simulink model "Landing"  (R2019a)
settings: Solver=ode14x  StartTime=0.0  StopTime=141  FixedStep=1/30  MaxStep=0.02  RelTol=1e-3
undefined symbols (not defined in the file): airport_elevation, con_init, con_trim, glideslope, h_flare, h_RWY, init_x_pos, Ka, Kq, Psi_RWY, RWY_vector, SS_long, tau, Th23, trim_elevator, trim_thrust
libraries: simulink_extras x13, simulink x3, aerolibfltsims x2, cstblocks x1, aerolibanimutils x1, aerolibatmos2 x1
settings Model: Creator=tblaha  LastModifiedBy=tblaha

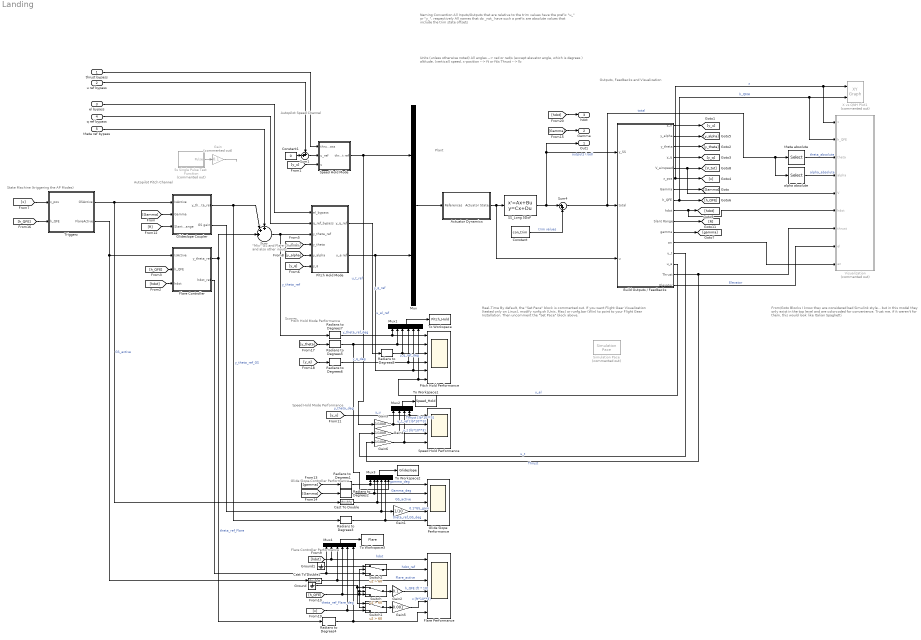
== system Landing ==
  note: Speed Hold Mode Performance
  note: Outputs, Feedbacks and Visualization
  note: Scopes
  note: Autopilot Speed Channel
  note: Autopilot Pitch Channel
  note: Plant
  note: State Machine (triggering the AP Modes)
  note: "Mix" GS and
      | Flare Channels
      | and also
      | other inputs
  note: Real-Time
      | By default, the "Set Pace" block is commented out.
      | If you want Flight Gear Visualization (tested only on Linux), modify runfg.sh (Unix, Mac) or runfg.bar (Win) to point to your Flight Gear Installation.
      | Then uncomment the "Set Pace" block above.
  note: From/Goto Blocks
      | I know they are considered bad Simulink style... but in this model they only exist in the top level and are colorcoded for convenience. Trust me, if it weren't for them, this would look like Italian Spaghetti
  note: Naming Convention
      | All Inputs/Outputs that are relative to the trim values have the prefix "u_" or "y_", respectively
      |
      | All names that do _not_ have such a prefix are absolute values that include the trim state offsets
  note: Units (unless otherwise noted)
      | All angles --> rad or rad/s (except elevator angle, which is degrees )
      | altitude, (vertical) speed, x-position --> ft or ft/s
      | Thrust --> lb
  note: Pitch Hold Mode Performance
  note: Flare Controller Performance
  note: Glide Slope Controller Performance
  thrust bypass : Inport
  u ref bypass : Inport  Port=2
  el bypass : Inport  Port=3
  q ref bypass : Inport  Port=4
  theta ref bypass : Inport  Port=5
  5s Single Pulse Test Function : Subsystem  Commented=on
  Actuator Dynamics : Subsystem
  Build Outputs / Feedbacks : Subsystem
  Cast To Double : DataTypeConversion  OutDataTypeStr=double
  Cast To Double1 : DataTypeConversion  OutDataTypeStr=double
  Constant : Constant  Value=con_trim
  Constant1 : Constant  Value=0
  Flare Controller : Subsystem
  Flare Performance : Scope  NumInputPorts=6
  Gain : Gain  Commented=on  Gain=0.1
  Gain1 : Gain  Gain=1/10
  Gain2 : Gain  Gain=0.1
  Gain3 : Gain  Gain=1/1000
  Gain4 : Gain  Gain=1/1000
  Gain5 : Gain  Gain=0.001
  Gain6 : Gain  Gain=1/1000
  Glide Slope Performance : Scope  NumInputPorts=5
  Glideslope Coupler : Subsystem
  Ground : Ground
  Ground1 : Ground
  Mux : Mux  Inputs=2
  Mux1 : Mux  Inputs=6
  Mux2 : Mux
  Mux3 : Mux  Inputs=6
  Mux4 : Mux  Inputs=6
  Pitch Hold Mode : Subsystem
  Pitch Hold Performance : Scope  NumInputPorts=6
  Radians to Degrees{1..8} (8 alike) : simulink_extras/Transformations/Radians to Degrees
  SS_Long 5DoF : StateSpace  A=SS_long.A  B=SS_long.B  C=SS_long.C  D=SS_long.D  InitialCondition=con_init
  Simulation Pace : aerolibanimutils/Simulation Pace  Commented=on  SimulationPace=1  SleepMode=Auto  OutputPaceError=off  SampleTime=1/30
  Speed Hold Mode : Subsystem
  Speed Hold Performance : Scope  NumInputPorts=4
  Sum : Sum  Inputs=+++||
  Sum1 : Sum  Inputs=++|
  Sum4 : Sum  Inputs=|++
  Switch : Switch  Criteria=u2 > Threshold  Threshold=60
  Switch1 : Switch  Criteria=u2 > Threshold  Threshold=60
  Switch2 : Switch  Criteria=u2 > Threshold  Threshold=60
  To Workspace : ToWorkspace  VariableName=Pitch_Hold  SampleTime=-1
  To Workspace1 : ToWorkspace  VariableName=Speed_Hold  SampleTime=-1
  To Workspace2 : ToWorkspace  VariableName=Glideslope  SampleTime=-1
  To Workspace3 : ToWorkspace  VariableName=Flare  SampleTime=-1
  Triggerz : Subsystem
  Visualization : Subsystem  Commented=on
  X vs QNH Plot1 : simulink/Sinks/XY Graph  Commented=on  xmin=-45000  xmax=5000  ymin=-100  ymax=2100  st=-1
  alpha absolute : Selector  InputPortWidth=5  IndexOptions=Index vector (dialog)  Indices=3  OutputSizes=1
  theta absolute : Selector  InputPortWidth=5  IndexOptions=Index vector (dialog)  Indices=4  OutputSizes=1
  Out1 : Outport
  Gamma : Outport  Port=2
  hdot : Outport  Port=3
  wires:
  Pitch Hold Mode/2(u_e ref) -> Mux/2, Mux1/5, Pitch Hold Performance/5  "u_el_ref"
  Speed Hold Mode/1(thrust ref) -> Mux/1, Gain3/1  "u_t_ref"
  [y_u] -> Speed Hold Mode/3(u)
  SS_Long 5DoF/1 -> Build Outputs / Feedbacks/1(y_SS), Out1/1, Sum4/1  "outputs (rad)"
  Build Outputs / Feedbacks/7(Gamma) -> [Gamma]
  Build Outputs / Feedbacks/11(gamma) -> [gamma]
  Build Outputs / Feedbacks/3(y_theta) -> [y_theta]
  Mux/1 -> Actuator Dynamics/1(References)
  Actuator Dynamics/1(Actuator States) -> SS_Long 5DoF/1, Build Outputs / Feedbacks/3(u)
  Build Outputs / Feedbacks/4(y_q) -> [y_q]
  Constant/1 -> Sum4/2  "trim values"
  Build Outputs / Feedbacks/1(y_u) -> [y_u]
  Build Outputs / Feedbacks/2(y_alpha) -> [y_alpha]
  Build Outputs / Feedbacks/10(Slant Range) -> [R]
  [x] -> Triggerz/1(x_pos)
  [h_QFE] -> Triggerz/2(h_QFE)
  [Gamma] -> Glideslope Coupler/2(Gamma)
  [R] -> Glideslope Coupler/3(SlantRange)
  Glideslope Coupler/1(y_theta_ref) -> Radians to Degrees3/1, Sum/2  "y_theta_ref_GS"
  [y_theta] -> Pitch Hold Mode/4(y_theta)
  [y_alpha] -> Pitch Hold Mode/5(y_alpha)
  [y_q] -> Pitch Hold Mode/6(y_q)
  [hdot] -> Flare Controller/3(hdot)
  [h_QFE] -> Flare Controller/2(h_QFE)
  5s Single Pulse Test Function/1(Pulse) -> Gain/1
  Build Outputs / Feedbacks/12(an) -> Visualization/9(an)
  alpha absolute/1 -> Visualization/4(alpha)  "alpha_absolute"
  Build Outputs / Feedbacks/9(hdot) -> Visualization/6(hdot), [hdot]
  Sum4/1 -> theta absolute/1, alpha absolute/1, Build Outputs / Feedbacks/2(total)  "total"
  theta absolute/1 -> Visualization/3(theta)  "theta_absolute"
  Build Outputs / Feedbacks/16(Elevator) -> Visualization/8(el)  "Elevator"
  Build Outputs / Feedbacks/8(h_QFE) -> [h_QFE], Visualization/2(h_QFE), X vs QNH Plot1/2  "h_QNH"
  Build Outputs / Feedbacks/15(Thrust) -> Gain6/1, Visualization/7(thrust)  "Thrust"
  Build Outputs / Feedbacks/5(V_airspeed) -> Visualization/5(V), [V_tot]
  Build Outputs / Feedbacks/6(x_pos) -> [x], Visualization/1(x), X vs QNH Plot1/1  "x"
  Pitch Hold Mode/1(y_q_ref) -> Radians to Degrees8/1  "y_q_ref"
  Radians to Degrees4/1 -> Flare Performance/6, Mux4/6  "theta_ref_Flare_deg"
  Radians to Degrees2/1 -> Mux3/2, Glide Slope Performance/2  "Gamma_deg"
  Flare Controller/1(y_theta_ref) -> Sum/3, Radians to Degrees4/1  "theta_ref_Flare"
  Gain1/1 -> Glide Slope Performance/4  "0.1*GS_gain"
  [y_q] -> Radians to Degrees6/1
  Radians to Degrees1/1 -> Glide Slope Performance/1, Mux3/1  "gamma_deg"
  [h_QFE] -> Switch1/2, Switch2/2, Switch/2, Switch/3, Mux4/4
  [Gamma] -> Radians to Degrees2/1
  Flare Controller/2(hdot_ref) -> Mux4/1, Switch2/3
  Build Outputs / Feedbacks/14(u_e) -> Mux1/6, Pitch Hold Performance/6  "u_el"
  [y_theta] -> Radians to Degrees5/1
  [gamma] -> Radians to Degrees1/1
  [hdot] -> Mux4/2, Flare Performance/1  "hdot"
  Radians to Degrees6/1 -> Mux1/4, Pitch Hold Performance/4  "y_q_deg"
  Triggerz/1(GSActive) -> Glideslope Coupler/1(IsActive), Cast To Double/1  "GS_active"
  Radians to Degrees7/1 -> Mux1/1, Pitch Hold Performance/1  "y_theta_ref_deg"
  Radians to Degrees5/1 -> Mux3/6, Mux1/2, Pitch Hold Performance/2  "y_theta_deg"
  Radians to Degrees8/1 -> Mux1/3, Pitch Hold Performance/3  "y_q_ref_deg"
  Triggerz/2(FlareActive) -> Flare Controller/1(IsActive), Cast To Double1/1
  Glideslope Coupler/2(GS gain) -> Gain1/1, Mux3/4
  Radians to Degrees3/1 -> Glide Slope Performance/5, Mux3/5  "theta_ref_GS_deg"
  theta ref bypass/1 -> Sum/1
  Build Outputs / Feedbacks/13(u_t) -> Gain4/1  "u_t"
  [y_u] -> Mux2/4, Speed Hold Performance/1  "y_u"
  Gain3/1 -> Mux2/1, Speed Hold Performance/2  "u_t_ref [lb*10**3]"
  Gain4/1 -> Speed Hold Performance/3, Mux2/2  "u_t [lb*10**3]"
  Gain6/1 -> Mux2/3, Speed Hold Performance/4  "Thrust [lb*10**3]"
  q ref bypass/1 -> Pitch Hold Mode/2(q_ref_bypass)
  el bypass/1 -> Pitch Hold Mode/1(el_bypass)
  Sum1/1 -> Speed Hold Mode/2(u_ref)
  u ref bypass/1 -> Sum1/1
  thrust bypass/1 -> Speed Hold Mode/1(thrust bypass)
  [Gamma] -> Gamma/1
  Sum/1 -> Radians to Degrees7/1, Pitch Hold Mode/3(y_theta_ref)  "y_theta_ref"
  Gain/1 -> ?
  [hdot] -> hdot/1
  Switch/1 -> Gain2/1
  Ground/1 -> Switch/1, Switch1/1
  Gain2/1 -> Flare Performance/4  "h_QFE [ft * 10]"
  Switch1/1 -> Gain5/1
  Gain5/1 -> Flare Performance/5  "x [ft*10**3]"
  [x] -> Switch1/3, Mux4/5
  Switch2/1 -> Flare Performance/2  "hdot_ref"
  Ground1/1 -> Switch2/1
  Constant1/1 -> Sum1/2
  Mux1/1 -> To Workspace/1
  Mux2/1 -> To Workspace1/1
  Mux3/1 -> To Workspace2/1
  Mux4/1 -> To Workspace3/1
  Cast To Double/1 -> Glide Slope Performance/3, Mux3/3  "GS_active"
  Cast To Double1/1 -> Flare Performance/3, Mux4/3  "Flare_active"

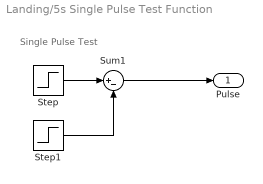
== system Landing/5s Single Pulse Test Function ==
  note: Single Pulse Test
  Step : Step  Time=5  SampleTime=0
  Step1 : Step  Time=10  SampleTime=0
  Sum1 : Sum  Inputs=|+-
  Pulse : Outport
  wires:
  Step/1 -> Sum1/1
  Step1/1 -> Sum1/2
  Sum1/1 -> Pulse/1

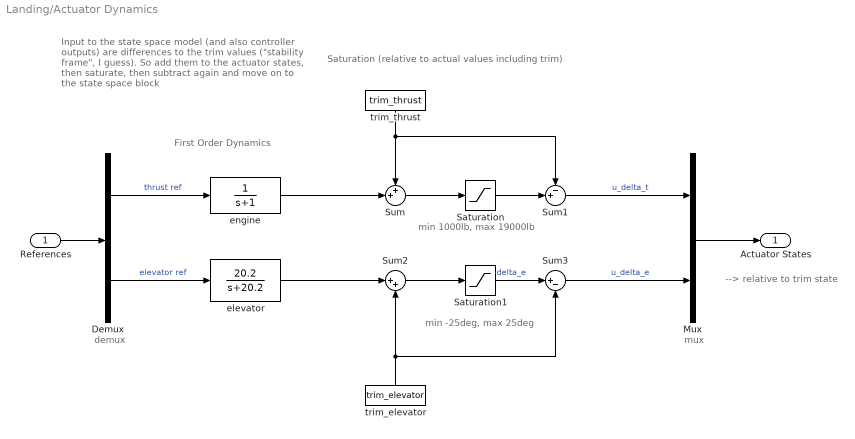
== system Landing/Actuator Dynamics ==
  note: --> relative to trim state
  note: Input to the state space model (and also controller outputs) are differences to the trim values ("stability frame", I guess). So add them to the actuator states, then saturate, then subtract again and move on to the state space block
  note: First Order Dynamics
  note: Saturation (relative to actual values including trim)
  note: demux
  note: min 1000lb, max 19000lb
  note: min -25deg, max 25deg
  note: mux
  References : Inport
  Demux : Demux  Outputs=2
  Mux : Mux  Inputs=2
  Saturation : Saturate  UpperLimit=19000  LowerLimit=1000
  Saturation1 : Saturate  UpperLimit=25  LowerLimit=-25
  Sum : Sum  Inputs=++|
  Sum1 : Sum  Inputs=-+|
  Sum2 : Sum  Inputs=|++
  Sum3 : Sum  Inputs=|+-
  elevator : TransferFcn  Numerator=[20.2]  Denominator=[1 20.2]
  engine : TransferFcn  Denominator=[1 1]
  trim_elevator : Constant  Value=trim_elevator
  trim_thrust : Constant  Value=trim_thrust
  Actuator States : Outport
  wires:
  References/1 -> Demux/1
  Demux/1 -> engine/1  "thrust ref"
  Demux/2 -> elevator/1  "elevator ref"
  engine/1 -> Sum/2
  Saturation/1 -> Sum1/2
  elevator/1 -> Sum2/1
  Saturation1/1 -> Sum3/1  "delta_e"
  Mux/1 -> Actuator States/1
  Sum/1 -> Saturation/1
  Sum1/1 -> Mux/1  "u_delta_t"
  trim_thrust/1 -> Sum1/1, Sum/1
  Sum2/1 -> Saturation1/1
  Sum3/1 -> Mux/2  "u_delta_e"
  trim_elevator/1 -> Sum3/2, Sum2/2

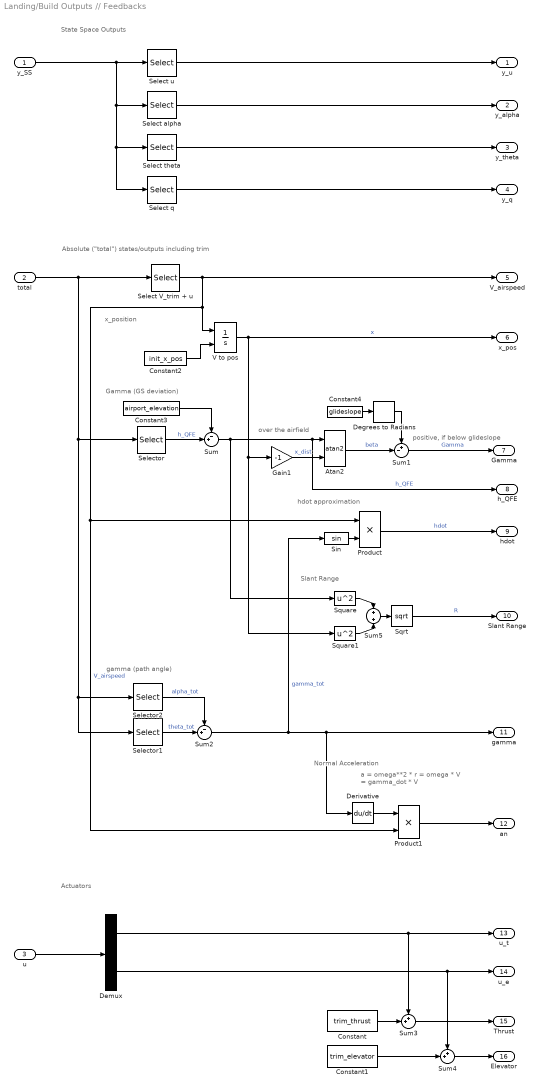
== system Landing/Build Outputs // Feedbacks ==
  note: hdot approximation
  note: Absolute ("total") states/outputs including trim
  note: State Space Outputs
  note: Actuators
  note: Slant Range
  note: gamma (path angle)
  note: positive, if
      | below glideslope
  note: Gamma (GS deviation)
  note: over the airfield
  note: x_position
  note: Normal Acceleration
  note: a = omega**2 * r
      |    = omega * V
      |    = gamma_dot * V
  y_SS : Inport
  total : Inport  Port=2
  u : Inport  Port=3
  Atan2 : Trigonometry  Operator=atan2
  Constant : Constant  Value=trim_thrust
  Constant1 : Constant  Value=trim_elevator
  Constant2 : Constant  Value=init_x_pos
  Constant3 : Constant  Value=airport_elevation
  Constant4 : Constant  Value=glideslope
  Degrees to Radians : simulink_extras/Transformations/Degrees to Radians
  Demux : Demux  Outputs=2
  Derivative : Derivative
  Gain1 : Gain  Gain=-1
  Product : Product
  Product1 : Product
  Select V_trim + u : Selector  InputPortWidth=5  IndexOptions=Index vector (dialog)  Indices=[2]  OutputSizes=1
  Select alpha : Selector  InputPortWidth=5  IndexOptions=Index vector (dialog)  Indices=3  OutputSizes=1
  Select q : Selector  InputPortWidth=5  IndexOptions=Index vector (dialog)  Indices=5  OutputSizes=1
  Select theta : Selector  InputPortWidth=5  IndexOptions=Index vector (dialog)  Indices=4  OutputSizes=1
  Select u : Selector  InputPortWidth=5  IndexOptions=Index vector (dialog)  Indices=[2]  OutputSizes=1
  Selector : Selector  InputPortWidth=5  IndexOptions=Index vector (dialog)  Indices=1  OutputSizes=1
  Selector1 : Selector  InputPortWidth=5  IndexOptions=Index vector (dialog)  Indices=4  OutputSizes=1
  Selector2 : Selector  InputPortWidth=5  IndexOptions=Index vector (dialog)  Indices=3  OutputSizes=1
  Sin : Trigonometry
  Sqrt : Sqrt  SaturateOnIntegerOverflow=on
  Square : Math  Operator=square  SaturateOnIntegerOverflow=on
  Square1 : Math  Operator=square  SaturateOnIntegerOverflow=on
  Sum : Sum  Inputs=-+|
  Sum1 : Sum  Inputs=+-|
  Sum2 : Sum  Inputs=-+|
  Sum3 : Sum  Inputs=++|
  Sum4 : Sum  Inputs=++|
  Sum5 : Sum
  V to pos : Integrator  InitialConditionSource=external
  y_u : Outport
  y_alpha : Outport  Port=2
  y_theta : Outport  Port=3
  y_q : Outport  Port=4
  V_airspeed : Outport  Port=5
  x_pos : Outport  Port=6
  Gamma : Outport  Port=7
  h_QFE : Outport  Port=8
  hdot : Outport  Port=9
  Slant Range : Outport  Port=10
  gamma : Outport  Port=11
  an : Outport  Port=12
  u_t : Outport  Port=13
  u_e : Outport  Port=14
  Thrust : Outport  Port=15
  Elevator : Outport  Port=16
  wires:
  Atan2/1 -> Sum1/2  "beta"
  Constant2/1 -> V to pos/2
  V to pos/1 -> x_pos/1, Gain1/1, Square1/1  "x"
  total/1 -> Select V_trim + u/1, Selector/1, Selector2/1, Selector1/1
  y_SS/1 -> Select q/1, Select theta/1, Select alpha/1, Select u/1
  Sum/1 -> Atan2/1, h_QFE/1, Square/1  "h_QFE"
  Square/1 -> Sum5/1
  Select q/1 -> y_q/1
  Square1/1 -> Sum5/2
  Constant3/1 -> Sum/1
  Select theta/1 -> y_theta/1
  Selector/1 -> Sum/2  "h_QFE"
  Sum1/1 -> Gamma/1  "Gamma"
  Selector2/1 -> Sum2/1  "alpha_tot"
  Sum2/1 -> Derivative/1, gamma/1, Sin/1  "gamma_tot"
  Sqrt/1 -> Slant Range/1  "R"
  Select alpha/1 -> y_alpha/1
  Selector1/1 -> Sum2/2  "theta_tot"
  Gain1/1 -> Atan2/2  "x_dist"
  Sum5/1 -> Sqrt/1
  Select V_trim + u/1 -> Product/1, Product1/2, V to pos/1, V_airspeed/1  "V_airspeed"
  Degrees to Radians/1 -> Sum1/1
  Constant4/1 -> Degrees to Radians/1
  Select u/1 -> y_u/1
  u/1 -> Demux/1
  Demux/1 -> u_t/1, Sum3/1
  Demux/2 -> u_e/1, Sum4/1
  Sum3/1 -> Thrust/1
  Constant/1 -> Sum3/2
  Sum4/1 -> Elevator/1
  Constant1/1 -> Sum4/2
  Sin/1 -> Product/2
  Product/1 -> hdot/1  "hdot"
  Derivative/1 -> Product1/1
  Product1/1 -> an/1

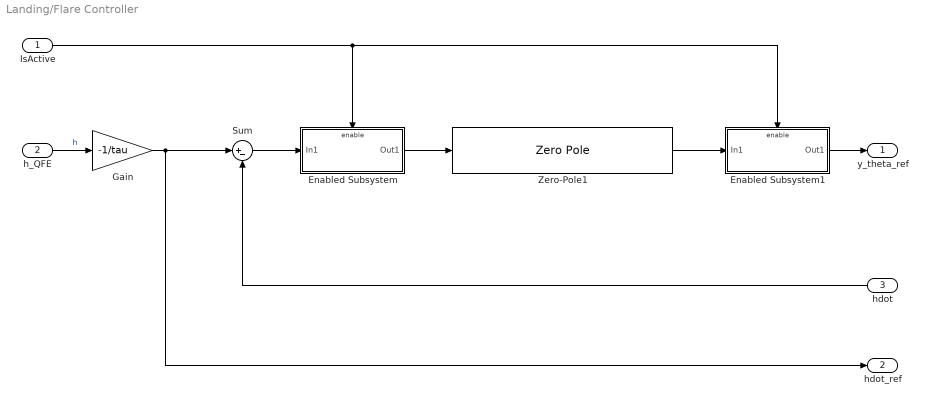
== system Landing/Flare Controller ==
  IsActive : Inport
  h_QFE : Inport  Port=2
  hdot : Inport  Port=3
  Enabled Subsystem : Subsystem  TreatAsAtomicUnit=on
  Enabled Subsystem1 : Subsystem  TreatAsAtomicUnit=on
  Gain : Gain  Gain=-1/tau
  Sum : Sum  Inputs=|+-
  Zero-Pole1 : ZeroPole  Zeros=[-0.23]  Poles=[0]  Gain=[0.01]
  y_theta_ref : Outport
  hdot_ref : Outport  Port=2
  wires:
  Gain/1 -> hdot_ref/1, Sum/1
  hdot/1 -> Sum/2
  IsActive/1 -> Enabled Subsystem/Enable, Enabled Subsystem1/Enable
  Sum/1 -> Enabled Subsystem/1(In1)
  Enabled Subsystem/1(Out1) -> Zero-Pole1/1
  h_QFE/1 -> Gain/1  "h"
  Enabled Subsystem1/1(Out1) -> y_theta_ref/1
  Zero-Pole1/1 -> Enabled Subsystem1/1(In1)

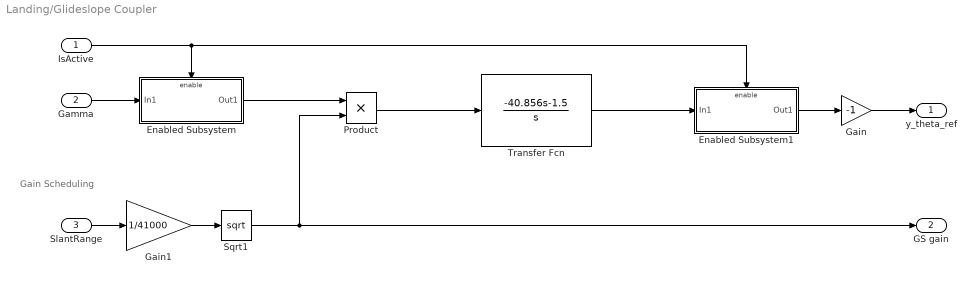
== system Landing/Glideslope Coupler ==
  note: Gain Scheduling
  IsActive : Inport
  Gamma : Inport  Port=2
  SlantRange : Inport  Port=3
  Enabled Subsystem : Subsystem  TreatAsAtomicUnit=on
  Enabled Subsystem1 : Subsystem  TreatAsAtomicUnit=on
  Gain : Gain  Gain=-1
  Gain1 : Gain  Gain=1/41000
  Product : Product
  Sqrt1 : Sqrt  SaturateOnIntegerOverflow=on
  Transfer Fcn : TransferFcn  Numerator=[-40.856 -1.5]  Denominator=[1 0]
  y_theta_ref : Outport
  GS gain : Outport  Port=2
  wires:
  Gamma/1 -> Enabled Subsystem/1(In1)
  IsActive/1 -> Enabled Subsystem1/Enable, Enabled Subsystem/Enable
  Enabled Subsystem1/1(Out1) -> Gain/1
  Transfer Fcn/1 -> Enabled Subsystem1/1(In1)
  Gain/1 -> y_theta_ref/1
  Gain1/1 -> Sqrt1/1
  SlantRange/1 -> Gain1/1
  Enabled Subsystem/1(Out1) -> Product/1
  Product/1 -> Transfer Fcn/1
  Sqrt1/1 -> Product/2, GS gain/1

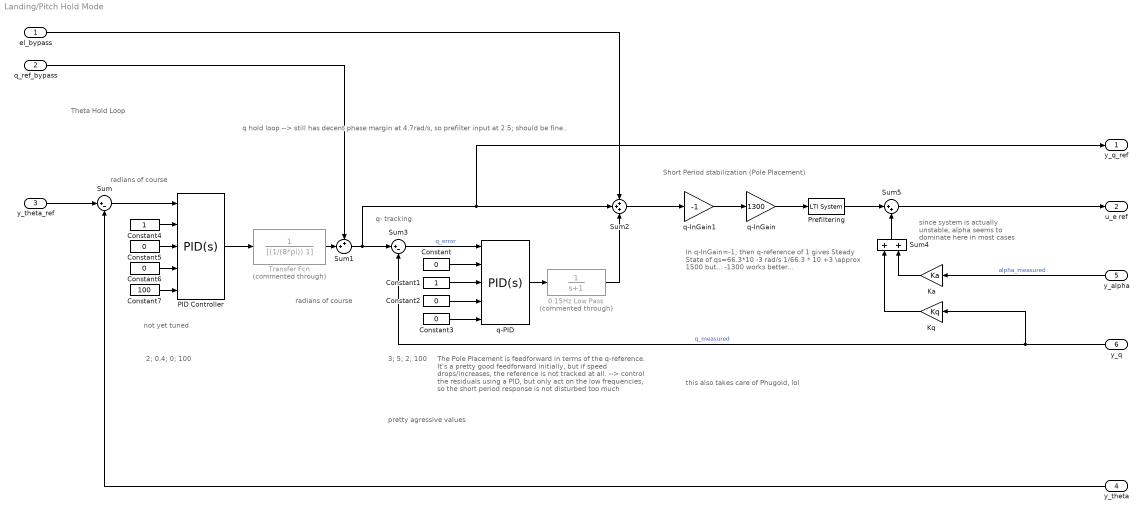
== system Landing/Pitch Hold Mode ==
  note: Theta Hold Loop
  note: not yet tuned
  note: 2;
      | 0.4;
      | 0;
      | 100
  note: this also takes care of Phugoid, lol
  note: since system is actually unstable, alpha seems to dominate here in most cases
  note: Short Period stabilization (Pole Placement)
  note: q- tracking
  note: The Pole Placement is feedforward in terms of the q-reference. It's a pretty good feedforward initially, but if speed drops/increases, the reference is not tracked at all. --> control the residuals using a PID, but only act on the low frequencies, so the short period response is not disturbed too much
  note: In q-InGain=-1; then q-reference of 1 gives
      |                          Steady State of qs=66.3*10 -3 rad/s
      | 			   1/66.3 * 10 +3 \approx 1500
      | but... -1300 works better...
  note: radians of course
  note: radians of course
  note: 3;
      | 5;
      | 2;
      | 100
  note: q hold loop --> still has decent phase margin at 4.7rad/s, so prefilter input at 2.5; should be fine..
  note: pretty agressive values
  el_bypass : Inport
  q_ref_bypass : Inport  Port=2
  y_theta_ref : Inport  Port=3
  y_theta : Inport  Port=4
  y_alpha : Inport  Port=5
  y_q : Inport  Port=6
  0.15Hz Low Pass : TransferFcn  Commented=through  Denominator=[1 1]
  Constant{,2..3,5..6} (5 alike) : Constant  Value=0
  Constant1 : Constant
  Constant4 : Constant
  Constant7 : Constant  Value=100
  Ka : Gain  Gain=Ka
  Kq : Gain  Gain=Kq
  PID Controller : simulink/Continuous/PID Controller  Controller=PID  Form=Ideal  TimeDomain=Continuous-time  SampleTime=-1  IntegratorMethod=Forward Euler  FilterMethod=Forward Euler  ControllerParametersSource=external  P=1  I=2  D=0.1  UseFilter=on  N=100  TunerSelectOption=Transfer Function Based (PID Tuner App)  InitialConditionSource=internal  InitialConditionForIntegrator=0  InitialConditionForFilter=0  DifferentiatorICPrevScaledInput=0  ExternalReset=none  TrackingMode=off  Kt=1  LimitOutput=off  UpperSaturationLimit=inf  LowerSaturationLimit=-inf  LinearizeAsGain=on  AntiWindupMode=none  Kb=1  POutMin=[]  POutMax=[]  IOutMin=[]  IOutMax=[]  DOutMin=[]  DOutMax=[]  NOutMin=[]  NOutMax=[]  SumOutMin=[]  SumOutMax=[]  SaturationOutMin=[]  SaturationOutMax=[]  PParamMin=[]  PParamMax=[]  IParamMin=[]  IParamMax=[]  DParamMin=[]  DParamMax=[]  NParamMin=[]  NParamMax=[]  KbParamMin=[]  KbParamMax=[]  KtParamMin=[]  KtParamMax=[]  KbOutMin=[]  KbOutMax=[]  KtOutMin=[]  KtOutMax=[]  IntegratorOutMin=[]  IntegratorOutMax=[]  FilterOutMin=[]  FilterOutMax=[]  SumI1OutMin=[]  SumI1OutMax=[]  SumI2OutMin=[]  SumI2OutMax=[]  SumI3OutMin=[]  SumI3OutMax=[]  SumI4OutMin=[]  SumI4OutMax=[]  SumDOutMin=[]  SumDOutMax=[]  DifferentiatorOutMin=[]  DifferentiatorOutMax=[]  FilterDiffOutCoefMin=[]  FilterDiffOutCoefMax=[]  ReciprocalOutMin=[]  ReciprocalOutMax=[]  SumDenOutMin=[]  SumDenOutMax=[]  SumNumOutMin=[]  SumNumOutMax=[]  DivideOutMin=[]  DivideOutMax=[]  IntegratorContinuousStateAttributes=''  IntegratorStateMustResolveToSignalObject=off  IntegratorRTWStateStorageClass=Auto  FilterContinuousStateAttributes=''  FilterStateMustResolveToSignalObject=off  FilterRTWStateStorageClass=Auto  ParallelPVariant=Passthrough  IdealPVariant=ExternalParameters  IVariant=ExternalParameters  DVariant=ExternalParameters  IntegratorVariant=Continuous  SatVariant=Disabled  AWVariant=Passthrough  PCopyVariant=Disabled  TRVariant=Disabled  FdbkBlocksVariant=Forward  IdealPFdbkVariant=Disabled  SatFdbkVariant=Disabled  DerivativeFilterVariant=ContFilter  NVariant=ExternalParameters  NCopyVariant=Disabled  FilterICVariant=InternalICsFilter  IntegratorICVariant=InternalICs  ExternalResetVariant=Disabled  TRSumVariant=Passthrough  SumFdbkVariant=Disabled  SumVariant=Sum_PID
  Prefiltering : cstblocks/LTI System  sys=LL_filt  IC=[]
  Sum : Sum  Inputs=|+-
  Sum1 : Sum  Inputs=++|
  Sum2 : Sum  Inputs=+++
  Sum3 : Sum  Inputs=|+-
  Sum4 : Sum
  Sum5 : Sum  Inputs=|++
  Transfer Fcn : TransferFcn  Commented=through  Denominator=[(1/(8*pi)) 1]
  q-InGain : Gain  Gain=1300
  q-InGain1 : Gain  Gain=-1
  q-PID : simulink/Continuous/PID Controller  Controller=PID  Form=Parallel  TimeDomain=Continuous-time  SampleTime=-1  IntegratorMethod=Forward Euler  FilterMethod=Forward Euler  ControllerParametersSource=external  P=1  I=0  D=0  UseFilter=on  N=100  TunerSelectOption=Transfer Function Based (PID Tuner App)  InitialConditionSource=internal  InitialConditionForIntegrator=0  InitialConditionForFilter=0  DifferentiatorICPrevScaledInput=0  ExternalReset=none  TrackingMode=off  Kt=1  LimitOutput=off  UpperSaturationLimit=inf  LowerSaturationLimit=-inf  LinearizeAsGain=on  AntiWindupMode=none  Kb=1  POutMin=[]  POutMax=[]  IOutMin=[]  IOutMax=[]  DOutMin=[]  DOutMax=[]  NOutMin=[]  NOutMax=[]  SumOutMin=[]  SumOutMax=[]  SaturationOutMin=[]  SaturationOutMax=[]  PParamMin=[]  PParamMax=[]  IParamMin=[]  IParamMax=[]  DParamMin=[]  DParamMax=[]  NParamMin=[]  NParamMax=[]  KbParamMin=[]  KbParamMax=[]  KtParamMin=[]  KtParamMax=[]  KbOutMin=[]  KbOutMax=[]  KtOutMin=[]  KtOutMax=[]  IntegratorOutMin=[]  IntegratorOutMax=[]  FilterOutMin=[]  FilterOutMax=[]  SumI1OutMin=[]  SumI1OutMax=[]  SumI2OutMin=[]  SumI2OutMax=[]  SumI3OutMin=[]  SumI3OutMax=[]  SumI4OutMin=[]  SumI4OutMax=[]  SumDOutMin=[]  SumDOutMax=[]  DifferentiatorOutMin=[]  DifferentiatorOutMax=[]  FilterDiffOutCoefMin=[]  FilterDiffOutCoefMax=[]  ReciprocalOutMin=[]  ReciprocalOutMax=[]  SumDenOutMin=[]  SumDenOutMax=[]  SumNumOutMin=[]  SumNumOutMax=[]  DivideOutMin=[]  DivideOutMax=[]  IntegratorContinuousStateAttributes=''  IntegratorStateMustResolveToSignalObject=off  IntegratorRTWStateStorageClass=Auto  FilterContinuousStateAttributes=''  FilterStateMustResolveToSignalObject=off  FilterRTWStateStorageClass=Auto  ParallelPVariant=ExternalParameters  IdealPVariant=Disabled  IVariant=ExternalParameters  DVariant=ExternalParameters  IntegratorVariant=Continuous  SatVariant=Disabled  AWVariant=Passthrough  PCopyVariant=Disabled  TRVariant=Disabled  FdbkBlocksVariant=Forward  IdealPFdbkVariant=Disabled  SatFdbkVariant=Disabled  DerivativeFilterVariant=ContFilter  NVariant=ExternalParameters  NCopyVariant=Disabled  FilterICVariant=InternalICsFilter  IntegratorICVariant=InternalICs  ExternalResetVariant=Disabled  TRSumVariant=Passthrough  SumFdbkVariant=Disabled  SumVariant=Sum_PID
  y_q_ref : Outport
  u_e ref : Outport  Port=2
  wires:
  Sum/1 -> PID Controller/1
  y_theta/1 -> Sum/2
  y_q/1 -> Sum3/2, Kq/1  "q_measured"
  y_alpha/1 -> Ka/1  "alpha_measured"
  Sum5/1 -> u_e ref/1
  q-PID/1 -> 0.15Hz Low Pass/1
  Constant/1 -> q-PID/2
  Constant1/1 -> q-PID/3
  Constant3/1 -> q-PID/5
  Constant2/1 -> q-PID/4
  Sum3/1 -> q-PID/1  "q_error"
  Sum4/1 -> Sum5/2
  Sum2/1 -> q-InGain1/1
  Prefiltering/1 -> Sum5/1
  Kq/1 -> Sum4/1
  q-InGain/1 -> Prefiltering/1
  Ka/1 -> Sum4/2
  Constant4/1 -> PID Controller/2
  Constant5/1 -> PID Controller/3
  Constant6/1 -> PID Controller/4
  Constant7/1 -> PID Controller/5
  PID Controller/1 -> Transfer Fcn/1
  q-InGain1/1 -> q-InGain/1
  y_theta_ref/1 -> Sum/1
  Sum1/1 -> Sum2/2, y_q_ref/1, Sum3/1
  Transfer Fcn/1 -> Sum1/2
  q_ref_bypass/1 -> Sum1/1
  el_bypass/1 -> Sum2/1
  0.15Hz Low Pass/1 -> Sum2/3

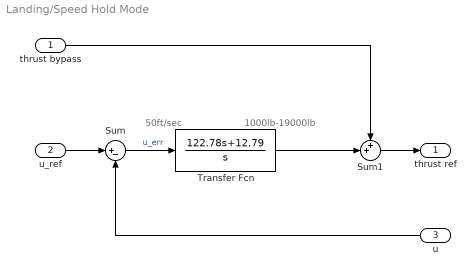
== system Landing/Speed Hold Mode ==
  note: 1000lb-19000lb
  note: 50ft/sec
  thrust bypass : Inport
  u_ref : Inport  Port=2
  u : Inport  Port=3
  Sum : Sum  Inputs=|+-
  Sum1 : Sum  Inputs=++|
  Transfer Fcn : TransferFcn  Numerator=[122.78 12.79]  Denominator=[1 0]
  thrust ref : Outport
  wires:
  u_ref/1 -> Sum/1
  u/1 -> Sum/2
  Sum1/1 -> thrust ref/1
  thrust bypass/1 -> Sum1/1
  Sum/1 -> Transfer Fcn/1  "u_err"
  Transfer Fcn/1 -> Sum1/2

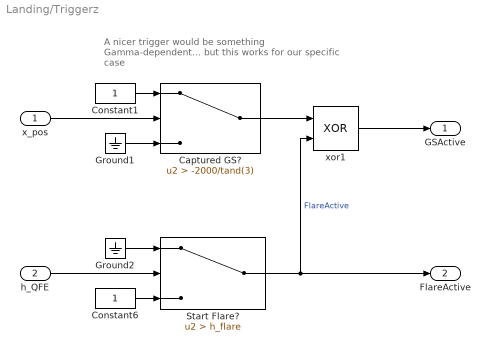
== system Landing/Triggerz ==
  note: A nicer trigger would be something Gamma-dependent... but this works for our specific case
  x_pos : Inport
  h_QFE : Inport  Port=2
  Captured GS? : Switch  Criteria=u2 > Threshold  Threshold=-2000/tand(3)
  Constant1 : Constant
  Constant6 : Constant
  Ground1 : Ground
  Ground2 : Ground
  Start Flare? : Switch  Criteria=u2 > Threshold  Threshold=h_flare
  xor1 : Logic  Operator=XOR  IconShape=distinctive  AllPortsSameDT=off  OutDataTypeStr=boolean
  GSActive : Outport
  FlareActive : Outport  Port=2
  wires:
  Ground2/1 -> Start Flare?/1
  Constant1/1 -> Captured GS?/1
  Start Flare?/1 -> FlareActive/1, xor1/2  "FlareActive"
  xor1/1 -> GSActive/1
  Ground1/1 -> Captured GS?/3
  h_QFE/1 -> Start Flare?/2
  Captured GS?/1 -> xor1/1
  x_pos/1 -> Captured GS?/2
  Constant6/1 -> Start Flare?/3

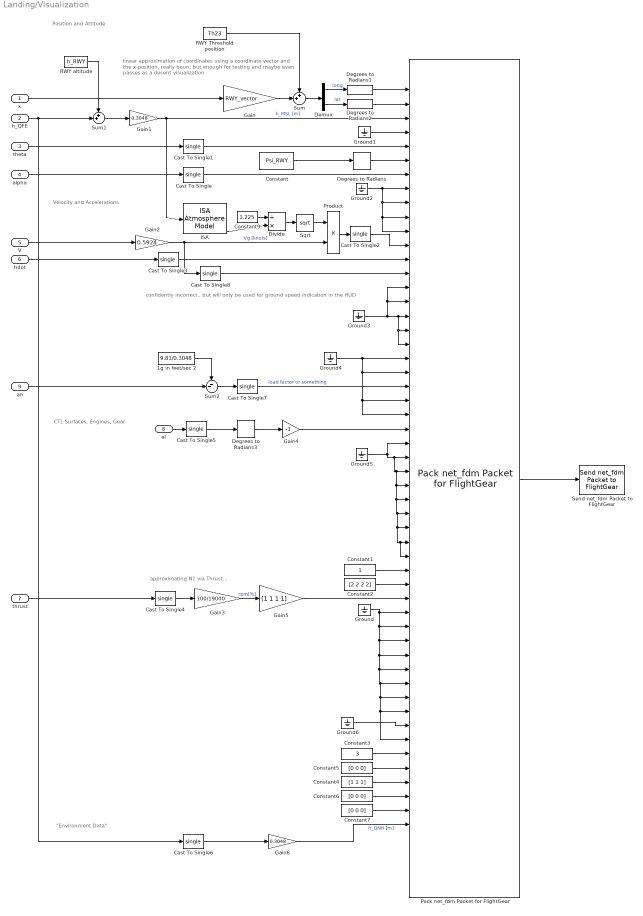
== system Landing/Visualization ==
  note: "Environment Data"
  note: CTL Surfaces, Engines, Gear
  note: Velocity and Accelerations
  note: Position and Attitude
  note: confidently incorrect.. but will only be used for ground speed indication in the HUD
  note: approximating N1 via Thrust...
  note: linear approximation of coordinates using a coordinate vector and the x-position, really beun; but enough for testing and maybe even passes as a decent visualization
  x : Inport
  h_QFE : Inport  Port=2
  theta : Inport  Port=3
  alpha : Inport  Port=4
  V : Inport  Port=5
  hdot : Inport  Port=6
  thrust : Inport  Port=7
  el : Inport  Port=8
  an : Inport  Port=9
  1g in feet/sec 2 : Constant  Value=9.81/0.3048
  Cast To Single{,1..8} (9 alike) : DataTypeConversion  OutDataTypeStr=single
  Constant : Constant  Value=Psi_RWY  OutDataTypeStr=single
  Constant1 : Constant  OutDataTypeStr=uint32
  Constant2 : Constant  Value=[2 2 2 2]  OutDataTypeStr=uint32
  Constant3 : Constant  Value=3  OutDataTypeStr=uint32
  Constant4 : Constant  Value=[1 1 1]  OutDataTypeStr=single
  Constant5 : Constant  Value=[0 0 0]  OutDataTypeStr=uint32
  Constant6 : Constant  Value=[0 0 0]  OutDataTypeStr=single
  Constant7 : Constant  Value=[0 0 0]  OutDataTypeStr=single
  Constant9 : Constant  Value=1.225
  Degrees to Radians{,1..3} (4 alike) : simulink_extras/Transformations/Degrees to Radians
  Demux : Demux  Outputs=2
  Divide : Product  Inputs=/*
  Gain : Gain  Gain=RWY_vector
  Gain1 : Gain  Gain=0.3048
  Gain2 : Gain  Gain=0.5924
  Gain3 : Gain  Gain=100/19000
  Gain4 : Gain  Gain=-1
  Gain5 : Gain  Gain=[1 1 1 1]
  Gain6 : Gain  Gain=0.3048
  Ground{,1..6} (7 alike) : Ground
  ISA : aerolibatmos2/ISA Atmosphere Model  custom=off  g=9.80665  gamma=1.4  R=287.0531  L=0.0065  h_trop=11000  h_strat=20000  rho0=1.225  P0=101325  T0=288.15  h0=0
      settings: SourceProductName=Aerospace Blockset
  Pack net_fdm Packet for FlightGear : aerolibfltsims/Pack net_fdm Packet for FlightGear  FlightGearVersion=v2018.2  ShowPositionAttitudeInputs=on  ShowVelocityAccelerationInputs=on  ShowControlSurfacePositionInputs=on  ShowEngineFuelInputs=on  ShowLandingGearInputs=on  ShowEnvironmentInputs=on  SampleTime=1/30  packetVersion=24
      settings: SourceProductName=Aerospace Blockset  SourceProductBaseCode=AE
  Product : Product
  RWY Threshold position : Constant  Value=Th23  OutDataTypeStr=double
  RWY altitude : Constant  Value=h_RWY  OutDataTypeStr=double
  Send net_fdm Packet to FlightGear : aerolibfltsims/Send net_fdm Packet to FlightGear  DestinationIpAddress=127.0.0.1  DestinationPort=5502  LocalIpPort=-1  varLen=off  SampleTime=1/30
      settings: SourceProductName=Aerospace Blockset  SourceProductBaseCode=AE
  Sqrt : Sqrt  SaturateOnIntegerOverflow=on
  Sum : Sum  Inputs=++|
  Sum1 : Sum  Inputs=++|
  Sum2 : Sum  Inputs=--|
  wires:
  Gain/1 -> Sum/2
  RWY Threshold position/1 -> Sum/1
  Sum/1 -> Demux/1
  Demux/1 -> Degrees to Radians1/1  "long"
  Demux/2 -> Degrees to Radians2/1  "lat"
  Gain1/1 -> Pack net_fdm Packet for FlightGear/3, ISA/1  "h_MSL [m]"
  RWY altitude/1 -> Sum1/1
  Sum1/1 -> Gain1/1
  Degrees to Radians/1 -> Pack net_fdm Packet for FlightGear/6
  Ground1/1 -> Pack net_fdm Packet for FlightGear/4
  theta/1 -> Cast To Single1/1
  Constant/1 -> Degrees to Radians/1
  Pack net_fdm Packet for FlightGear/1 -> Send net_fdm Packet to FlightGear/1
  alpha/1 -> Cast To Single/1
  Ground2/1 -> Pack net_fdm Packet for FlightGear/9, Pack net_fdm Packet for FlightGear/11, Pack net_fdm Packet for FlightGear/10, Pack net_fdm Packet for FlightGear/8
  Gain2/1 -> Cast To Single8/1, Product/2  "Vg [knots]"
  hdot/1 -> Cast To Single3/1
  Ground4/1 -> Pack net_fdm Packet for FlightGear/20, Pack net_fdm Packet for FlightGear/21, Pack net_fdm Packet for FlightGear/24, Pack net_fdm Packet for FlightGear/23
  Constant1/1 -> Pack net_fdm Packet for FlightGear/35
  Constant2/1 -> Pack net_fdm Packet for FlightGear/36
  Gain3/1 -> Gain5/1  "rpm[%]"
  thrust/1 -> Cast To Single4/1
  Ground/1 -> Pack net_fdm Packet for FlightGear/47, Pack net_fdm Packet for FlightGear/45, Pack net_fdm Packet for FlightGear/44, Pack net_fdm Packet for FlightGear/43, Pack net_fdm Packet for FlightGear/42, Pack net_fdm Packet for FlightGear/41, Pack net_fdm Packet for FlightGear/40, Pack net_fdm Packet for FlightGear/39, Pack net_fdm Packet for FlightGear/38
  Constant3/1 -> Pack net_fdm Packet for FlightGear/48
  Constant5/1 -> Pack net_fdm Packet for FlightGear/49
  Constant4/1 -> Pack net_fdm Packet for FlightGear/50
  Constant6/1 -> Pack net_fdm Packet for FlightGear/51
  Constant7/1 -> Pack net_fdm Packet for FlightGear/52
  el/1 -> Cast To Single5/1
  Gain5/1 -> Pack net_fdm Packet for FlightGear/37
  Ground6/1 -> Pack net_fdm Packet for FlightGear/46
  Cast To Single/1 -> Pack net_fdm Packet for FlightGear/7
  Cast To Single1/1 -> Pack net_fdm Packet for FlightGear/5
  x/1 -> Gain/1
  h_QFE/1 -> Sum1/2, Cast To Single6/1
  Cast To Single4/1 -> Gain3/1
  V/1 -> Gain2/1
  Cast To Single3/1 -> Pack net_fdm Packet for FlightGear/13
  Cast To Single5/1 -> Degrees to Radians3/1
  Degrees to Radians1/1 -> Pack net_fdm Packet for FlightGear/1
  Degrees to Radians2/1 -> Pack net_fdm Packet for FlightGear/2
  Degrees to Radians3/1 -> Gain4/1
  Gain4/1 -> Pack net_fdm Packet for FlightGear/25
  Ground5/1 -> Pack net_fdm Packet for FlightGear/34, Pack net_fdm Packet for FlightGear/33, Pack net_fdm Packet for FlightGear/32, Pack net_fdm Packet for FlightGear/31, Pack net_fdm Packet for FlightGear/30, Pack net_fdm Packet for FlightGear/29, Pack net_fdm Packet for FlightGear/28, Pack net_fdm Packet for FlightGear/27, Pack net_fdm Packet for FlightGear/26
  Cast To Single6/1 -> Gain6/1
  Gain6/1 -> Pack net_fdm Packet for FlightGear/53  "h_QNH [m]"
  Cast To Single7/1 -> Pack net_fdm Packet for FlightGear/22  "load factor or something"
  an/1 -> Sum2/2
  1g in feet/sec 2/1 -> Sum2/1
  Sum2/1 -> Cast To Single7/1
  ISA/4 -> Divide/2
  Product/1 -> Cast To Single2/1
  Constant9/1 -> Divide/1
  Divide/1 -> Sqrt/1
  Sqrt/1 -> Product/1
  Cast To Single2/1 -> Pack net_fdm Packet for FlightGear/12
  Cast To Single8/1 -> Pack net_fdm Packet for FlightGear/14
  Ground3/1 -> Pack net_fdm Packet for FlightGear/16, Pack net_fdm Packet for FlightGear/15, Pack net_fdm Packet for FlightGear/19, Pack net_fdm Packet for FlightGear/18, Pack net_fdm Packet for FlightGear/17

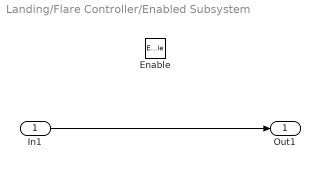
== system Landing/Flare Controller/Enabled Subsystem ==
  In1 : Inport
  Enable : EnablePort
  Out1 : Outport
  wires:
  In1/1 -> Out1/1

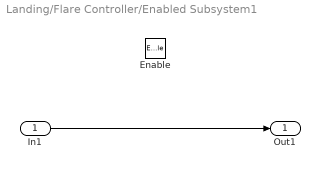
== system Landing/Flare Controller/Enabled Subsystem1 ==
  In1 : Inport
  Enable : EnablePort
  Out1 : Outport
  wires:
  In1/1 -> Out1/1

== system Landing/Glideslope Coupler/Enabled Subsystem ==
  In1 : Inport
  Enable : EnablePort
  Out1 : Outport
  wires:
  In1/1 -> Out1/1

== system Landing/Glideslope Coupler/Enabled Subsystem1 ==
  In1 : Inport
  Enable : EnablePort
  Out1 : Outport
  wires:
  In1/1 -> Out1/1
